simulink model "VTOL_sim"  (R2015a)
settings: Solver=ode45  StartTime=0.0  StopTime=10000  RelTol=1e-3
InitFcn:
  | param
undefined symbols (not defined in the file or in its folder): AP, drawVTOL, P
libraries: simulink x2
settings Model: Creator=beard  LastModifiedBy=beard
settings DataIOCC: SignalLoggingSaveFormat=ModelDataLogs
settings OptimizationCC: ExpressionDepthLimit=2147483647  InitFltsAndDblsToZero=on
settings DebuggingCC: UnderspecifiedInitializationDetection=Classic  MergeDetectMultiDrivingBlocksExec=none  SolverPrmCheckMsg=warning  FcnCallInpInsideContextMsg=UseLocalSettings  StateNameClashWarn=warning
settings GRTTargetCC: CombineOutputUpdateFcns=off  GRTInterface=on

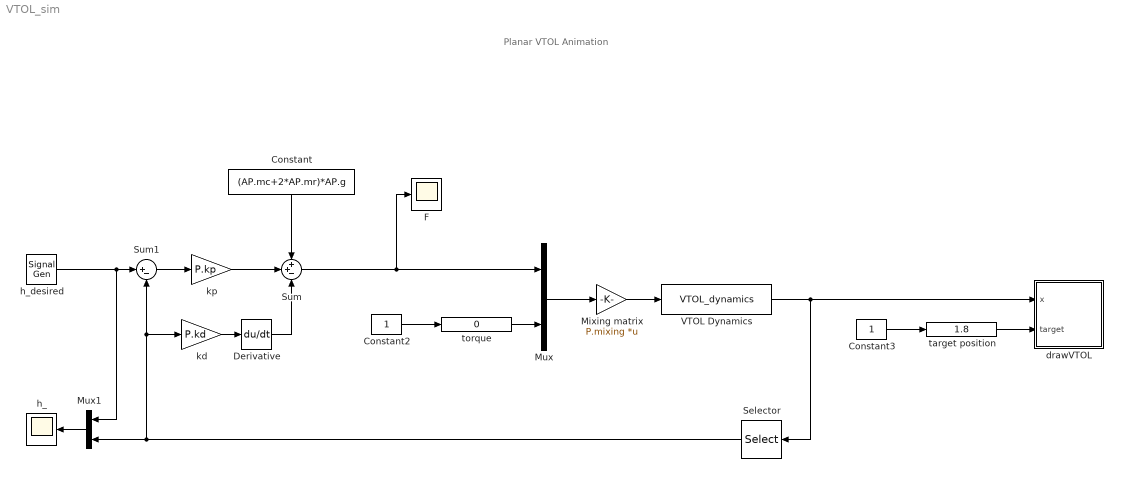
== system VTOL_sim ==
  note: Planar VTOL Animation
  Constant : Constant  Value=(AP.mc+2*AP.mr)*AP.g
  Constant2 : Constant
  Constant3 : Constant
  Derivative : Derivative
  F : Scope
      settings: TimeRange=58.5  YMin=12  YMax=20
  Mixing matrix : Gain  Gain=P.mixing  Multiplication=Matrix(K*u)
  Mux : Mux  Inputs=2
  Mux1 : Mux  Inputs=2
  Selector : Selector  InputPortWidth=3  Indices=[2]
  Sum : Sum  Inputs=++-
  Sum1 : Sum  Inputs=|+-
  VTOL Dynamics : S-Function  FunctionName=VTOL_dynamics  Parameters=AP
  drawVTOL : Subsystem
      mask Display: image(imread('tv.jpg'))
  h_ : Scope
      settings: TimeRange=100  YMin=-3.5  YMax=4
  h_desired : SignalGenerator  WaveForm=square  Amplitude=2.5  Frequency=.02
  kd : Gain  Gain=P.kd
  kp : Gain  Gain=P.kp
  target position : simulink/Math Operations/Slider Gain  low=-10  gain=1.8  high=50
  torque : simulink/Math Operations/Slider Gain  low=-1  gain=0  high=1
  wires:
  Constant2/1 -> torque/1
  torque/1 -> Mux/2
  Constant3/1 -> target position/1
  VTOL Dynamics/1 -> Selector/1, drawVTOL/1(x)
  target position/1 -> drawVTOL/2(target)
  Sum/1 -> Mux/1, F/1
  Sum1/1 -> kp/1
  h_desired/1 -> Sum1/1, Mux1/1
  Mux1/1 -> h_/1
  kp/1 -> Sum/2
  Constant/1 -> Sum/1
  kd/1 -> Derivative/1
  Derivative/1 -> Sum/3
  Mixing matrix/1 -> VTOL Dynamics/1
  Mux/1 -> Mixing matrix/1
  Selector/1 -> kd/1, Sum1/2, Mux1/2

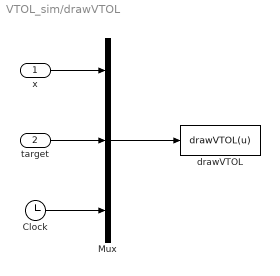
== system VTOL_sim/drawVTOL ==
  x : Inport
  target : Inport  Port=2
  Clock : Clock
  Mux : Mux  Inputs=3
  drawVTOL : MATLABFcn  MATLABFcn=drawVTOL(u)  OutputDimensions=0  SampleTime=0.1
  wires:
  Mux/1 -> drawVTOL/1
  x/1 -> Mux/1
  Clock/1 -> Mux/3
  target/1 -> Mux/2
